simulink model "test_newfft_fun2"  (Simulink 6.2)
settings: Solver=ode45  StartTime=0.0  StopTime=3200.0  RelTol=1e-3
libraries: xbsIndex_r3 x643, simulink x1
(part 4 of 10)

== system test_newfft_fun2/r2_dit_fft/r2_dit_stage_5 ==
  a_in : Inport  Port=1  LatchInput=off
  b_in : Inport  Port=2  LatchInput=off
  sync_in : Inport  Port=3  LatchInput=off
  biplex_commutator : Subsystem  mask(Biplex Commutator){log2_size=6, n_bits=12, use_bram=off}
      mask prompts: log2_size "Log2 Block Size"; n_bits "Bit Width"; use_bram "Use BRAM"
      mask help: The biplex commutator commutes the first half of the BloBhi input "block" with the last half of the AloAhi input "block". A "block" is 2^log2_size consecutive samples (i.e. always a power of 2). sync_in precedes the first data input sample by one clock cycle. Overall latency from sync_in to sync_out is 2^(log2_size-1)+1.
      settings: AttributesFormatString=|
      | size = 64
      | delay slr
      mask Help:
      | <pre>
      | Description::
      | 
      | The biplex commutator commutes the first half of the BloBhi input "block"  with the last half
      | of the AloAhi input "block".  A "block" is 2^log2_size consecutive samples (i.e. always a
      | power of 2).
      | 
      | sync_in precedes the first data input sample by one clock cycle.
      | sync_out precedes the corresponding output sample by one clock cycle.
      | Overall latency from sync_in to sync_out is 2^(N-1)+1.
      | 
      | Mask Parameters::
      | 
      | Log 2 Block Size (log2_size): The base-2 logarithm of the length of one complete input block.
      | This MUST be an integer because the current implementation requires that
      | the input block size MUST be a power of 2.  (aka "N")
      | 
      | Bit Width (n_bits): Specifies the width of the real/imaginary components.
      | Width of each component is assumed equal.
      | 
      | Use BRAM (use_bram): Check this checkbox to implement the internal delays using BRAM.
      | If unchecked, the internal delays will be implemented using SLR16 elements.
      | </pre>
  r2_butterfly : Subsystem  mask(Radix-2 Butterfly){n_bits=12, shift=0, quantization=Truncate, add_latency=1}
      mask prompts: n_bits "Bit Width In"; shift "Shift Bits"; add_latency "Adder Latency"
      mask help: The radix-2 butterfly produces a+b and a-b outputs for a and b inputs.
      settings: AttributesFormatString=shift 0
      mask Help:
      | <pre>
      | Description::
      | 
      | The radix-2 butterfly produces a+b and a-b outputs for a and b inputs.
      | The outputs are one bit wider than the inputs.
      | The output precision (i.e. the number of fractional bits) stays the same.
      | 
      | Mask Parameters::
      | 
      | Bit Width In (n_bits): Specifies the width of the real/imaginary components.
      | Width of each component is assumed equal.
      | 
      | Shift Bits (shift): Specifies how many bits to shift (down) by.  A positive value causes
      | the specified number of least significant bits to be dropped.  Usually zero or positive values
      | are used to permit or limit bit growth, but negative values can be used to induce bit growth.
      | 
      | Quantization (quantization): Specifies quantization handling (when shift bits > 0).
      | 
      | Adder Latency (add_latency): Latency to use for the underlying real adders.
      | </pre>
      mask StyleString: edit,edit,popup(Truncate|Round  (unbiased: +/- Inf)|Round  (unbiased: Even Values)),edit
  r2_twiddle : Subsystem  mask(Radix-2 General Twiddle Stage){n_stages=10, cur_stage=5, decimation=Time, n_bits=12, bin_pt=7, n_bits_w=8, use_bram=off, mult_latency=3, add_latency=1}
      mask prompts: n_stages "Total Stages"; cur_stage "Current Stage"; decimation "Decimation Mode"; n_bits "Number of Bits In/Out"; bin_pt "Binary Point In/Out"; n_bits_w "Twiddle Coefficient Bitwidth"; use_bram "Use BRAM For Twiddle Coefficients"; mult_latency "Multiplier Latency"; add_latency "Adder Latency"
      mask help: A general twiddle stage for radix-2 Fast Fourier Transforms. Can be used in Decimation in Time (i.e. twiddles before butterflies) or Decimation in Frequency (i.e. twiddles after butterflies) FFTs. Regardless of the decimation mode, the FFT is assumed to have inputs in normal order and outputs in bit-reversed order.
      settings: AttributesFormatString=16 twiddles in dist
      mask Help:
      | <pre>
      | Description::
      | 
      | A general twiddle stage for radix-2 Fast Fourier Transforms.
      | 
      | Can be used in  Decimation in Time (i.e. twiddles before butterflies) or Decimation in Frequency
      | (i.e. twiddles after butterflies) FFTs.  Regardless of the decimation mode, the FFT is assumed
      | to have inputs in normal order and outputs in bit-reversed order.
      | 
      | Input a_in is passed through unchanged to a_out, while input b is passed through to bw after
      | being "twiddled".  Since twiddling is effectively multiplication by a complex number with unity
      | magnitude, the bit respresentation of bw is the same as b (i.e. twiddling does not cause bit
      | growth).  Input a_in is assumed to have the same bit width as b.  Thus, a_in, a_out, b, and
      | bw all have the same bit representation.
      | 
      | Mask Parameters::
      | 
      | Total Stages (n_stages):  The number of total stages in the FFT.
      | The FFT will have 2^n_stages points.
      | 
      | Current Stage (cur_stage):  The number of the current stage for which this block should
      | generate twiddle coefficients.  Valid values are 3 through n_stages, inclusive.  Note that
      | stages are counted from 1 to n_stages for DIT (i.e. cur_stage==1 for the first stage) and
      | n_stages to 1 for DIF (i.e. cur_stage==1 for the last stage).
      | 
      | Decimation Mode (decimation): The decimation mode of the FFT.
      | 
      | Number of Bits In/Out (n_bits): Specifies the width of the real/imaginary
      | components of ports a_in, b, a_out, bw.  Assumed equal for both components.
      | 
      | Binary Point In/Out (bin_pt): Specifies the binary point position of the real/imaginary
      | components of ports a_in, b, a_out, bw.  Assumed equal for both components.
      | 
      | Twiddle Coefficient Bitwidth (n_bits_w): Specifies the width of the real/imaginary
      | components of the twiddle coefficients.  Assumed equal for both components.
      | 
      | Use BRAM for Twiddle Coefficients (use_bram): Check this checkbox to store twiddle
      | coefficients in BRAM.  If unchecked, the twiddle coefficients will be sored in distributed
      | memory (i.e. slices).
      | 
      | Multiplier Latency (mult_latency): Latency to use for the underlying real multipliers.
      | 
      | Adder Latency (add_latency): Latency to use for the underlying real adders.
      mask StyleString: edit,edit,popup(Time|Frequency),edit,edit,edit,checkbox,edit,edit
  a_out : Outport
  b_out : Outport  Port=2
  sync_out : Outport  Port=3
  wires:
  r2_butterfly/3(sync_out) -> sync_out/1
  r2_butterfly/2(a-b) -> b_out/1
  r2_butterfly/1(a+b) -> a_out/1
  sync_in/1 -> biplex_commutator/3(sync_in)
  b_in/1 -> biplex_commutator/2(BloBhi)
  a_in/1 -> biplex_commutator/1(AloAhi)
  biplex_commutator/3(sync_out) -> r2_twiddle/3(sync_in)
  biplex_commutator/2(AhiBhi) -> r2_twiddle/2(b)
  biplex_commutator/1(AloBlo) -> r2_twiddle/1(a_in)
  r2_twiddle/1(a_out) -> r2_butterfly/1(a)
  r2_twiddle/2(bw) -> r2_butterfly/2(b)
  r2_twiddle/3(sync_out) -> r2_butterfly/3(sync_in)

== system test_newfft_fun2/r2_dit_fft/r2_dit_stage_6 ==
  a_in : Inport  Port=1  LatchInput=off
  b_in : Inport  Port=2  LatchInput=off
  sync_in : Inport  Port=3  LatchInput=off
  biplex_commutator : Subsystem  mask(Biplex Commutator){log2_size=5, n_bits=13, use_bram=off}
      mask prompts: log2_size "Log2 Block Size"; n_bits "Bit Width"; use_bram "Use BRAM"
      mask help: The biplex commutator commutes the first half of the BloBhi input "block" with the last half of the AloAhi input "block". A "block" is 2^log2_size consecutive samples (i.e. always a power of 2). sync_in precedes the first data input sample by one clock cycle. Overall latency from sync_in to sync_out is 2^(log2_size-1)+1.
      settings: AttributesFormatString=|
      | size = 32
      | delay slr
      mask Help:
      | <pre>
      | Description::
      | 
      | The biplex commutator commutes the first half of the BloBhi input "block"  with the last half
      | of the AloAhi input "block".  A "block" is 2^log2_size consecutive samples (i.e. always a
      | power of 2).
      | 
      | sync_in precedes the first data input sample by one clock cycle.
      | sync_out precedes the corresponding output sample by one clock cycle.
      | Overall latency from sync_in to sync_out is 2^(N-1)+1.
      | 
      | Mask Parameters::
      | 
      | Log 2 Block Size (log2_size): The base-2 logarithm of the length of one complete input block.
      | This MUST be an integer because the current implementation requires that
      | the input block size MUST be a power of 2.  (aka "N")
      | 
      | Bit Width (n_bits): Specifies the width of the real/imaginary components.
      | Width of each component is assumed equal.
      | 
      | Use BRAM (use_bram): Check this checkbox to implement the internal delays using BRAM.
      | If unchecked, the internal delays will be implemented using SLR16 elements.
      | </pre>
  r2_butterfly : Subsystem  mask(Radix-2 Butterfly){n_bits=13, shift=0, quantization=Truncate, add_latency=1}
      mask prompts: n_bits "Bit Width In"; shift "Shift Bits"; add_latency "Adder Latency"
      mask help: The radix-2 butterfly produces a+b and a-b outputs for a and b inputs.
      settings: AttributesFormatString=shift 0
      mask Help:
      | <pre>
      | Description::
      | 
      | The radix-2 butterfly produces a+b and a-b outputs for a and b inputs.
      | The outputs are one bit wider than the inputs.
      | The output precision (i.e. the number of fractional bits) stays the same.
      | 
      | Mask Parameters::
      | 
      | Bit Width In (n_bits): Specifies the width of the real/imaginary components.
      | Width of each component is assumed equal.
      | 
      | Shift Bits (shift): Specifies how many bits to shift (down) by.  A positive value causes
      | the specified number of least significant bits to be dropped.  Usually zero or positive values
      | are used to permit or limit bit growth, but negative values can be used to induce bit growth.
      | 
      | Quantization (quantization): Specifies quantization handling (when shift bits > 0).
      | 
      | Adder Latency (add_latency): Latency to use for the underlying real adders.
      | </pre>
      mask StyleString: edit,edit,popup(Truncate|Round  (unbiased: +/- Inf)|Round  (unbiased: Even Values)),edit
  r2_twiddle : Subsystem  mask(Radix-2 General Twiddle Stage){n_stages=10, cur_stage=6, decimation=Time, n_bits=13, bin_pt=7, n_bits_w=8, use_bram=off, mult_latency=3, add_latency=1}
      mask prompts: n_stages "Total Stages"; cur_stage "Current Stage"; decimation "Decimation Mode"; n_bits "Number of Bits In/Out"; bin_pt "Binary Point In/Out"; n_bits_w "Twiddle Coefficient Bitwidth"; use_bram "Use BRAM For Twiddle Coefficients"; mult_latency "Multiplier Latency"; add_latency "Adder Latency"
      mask help: A general twiddle stage for radix-2 Fast Fourier Transforms. Can be used in Decimation in Time (i.e. twiddles before butterflies) or Decimation in Frequency (i.e. twiddles after butterflies) FFTs. Regardless of the decimation mode, the FFT is assumed to have inputs in normal order and outputs in bit-reversed order.
      settings: AttributesFormatString=32 twiddles in dist
      mask Help:
      | <pre>
      | Description::
      | 
      | A general twiddle stage for radix-2 Fast Fourier Transforms.
      | 
      | Can be used in  Decimation in Time (i.e. twiddles before butterflies) or Decimation in Frequency
      | (i.e. twiddles after butterflies) FFTs.  Regardless of the decimation mode, the FFT is assumed
      | to have inputs in normal order and outputs in bit-reversed order.
      | 
      | Input a_in is passed through unchanged to a_out, while input b is passed through to bw after
      | being "twiddled".  Since twiddling is effectively multiplication by a complex number with unity
      | magnitude, the bit respresentation of bw is the same as b (i.e. twiddling does not cause bit
      | growth).  Input a_in is assumed to have the same bit width as b.  Thus, a_in, a_out, b, and
      | bw all have the same bit representation.
      | 
      | Mask Parameters::
      | 
      | Total Stages (n_stages):  The number of total stages in the FFT.
      | The FFT will have 2^n_stages points.
      | 
      | Current Stage (cur_stage):  The number of the current stage for which this block should
      | generate twiddle coefficients.  Valid values are 3 through n_stages, inclusive.  Note that
      | stages are counted from 1 to n_stages for DIT (i.e. cur_stage==1 for the first stage) and
      | n_stages to 1 for DIF (i.e. cur_stage==1 for the last stage).
      | 
      | Decimation Mode (decimation): The decimation mode of the FFT.
      | 
      | Number of Bits In/Out (n_bits): Specifies the width of the real/imaginary
      | components of ports a_in, b, a_out, bw.  Assumed equal for both components.
      | 
      | Binary Point In/Out (bin_pt): Specifies the binary point position of the real/imaginary
      | components of ports a_in, b, a_out, bw.  Assumed equal for both components.
      | 
      | Twiddle Coefficient Bitwidth (n_bits_w): Specifies the width of the real/imaginary
      | components of the twiddle coefficients.  Assumed equal for both components.
      | 
      | Use BRAM for Twiddle Coefficients (use_bram): Check this checkbox to store twiddle
      | coefficients in BRAM.  If unchecked, the twiddle coefficients will be sored in distributed
      | memory (i.e. slices).
      | 
      | Multiplier Latency (mult_latency): Latency to use for the underlying real multipliers.
      | 
      | Adder Latency (add_latency): Latency to use for the underlying real adders.
      mask StyleString: edit,edit,popup(Time|Frequency),edit,edit,edit,checkbox,edit,edit
  a_out : Outport
  b_out : Outport  Port=2
  sync_out : Outport  Port=3
  wires:
  r2_butterfly/3(sync_out) -> sync_out/1
  r2_butterfly/2(a-b) -> b_out/1
  r2_butterfly/1(a+b) -> a_out/1
  sync_in/1 -> biplex_commutator/3(sync_in)
  b_in/1 -> biplex_commutator/2(BloBhi)
  a_in/1 -> biplex_commutator/1(AloAhi)
  biplex_commutator/3(sync_out) -> r2_twiddle/3(sync_in)
  biplex_commutator/2(AhiBhi) -> r2_twiddle/2(b)
  biplex_commutator/1(AloBlo) -> r2_twiddle/1(a_in)
  r2_twiddle/1(a_out) -> r2_butterfly/1(a)
  r2_twiddle/2(bw) -> r2_butterfly/2(b)
  r2_twiddle/3(sync_out) -> r2_butterfly/3(sync_in)

== system test_newfft_fun2/r2_dit_fft/r2_dit_stage_7 ==
  a_in : Inport  Port=1  LatchInput=off
  b_in : Inport  Port=2  LatchInput=off
  sync_in : Inport  Port=3  LatchInput=off
  biplex_commutator : Subsystem  mask(Biplex Commutator){log2_size=4, n_bits=14, use_bram=off}
      mask prompts: log2_size "Log2 Block Size"; n_bits "Bit Width"; use_bram "Use BRAM"
      mask help: The biplex commutator commutes the first half of the BloBhi input "block" with the last half of the AloAhi input "block". A "block" is 2^log2_size consecutive samples (i.e. always a power of 2). sync_in precedes the first data input sample by one clock cycle. Overall latency from sync_in to sync_out is 2^(log2_size-1)+1.
      settings: AttributesFormatString=|
      | size = 16
      | delay slr
      mask Help:
      | <pre>
      | Description::
      | 
      | The biplex commutator commutes the first half of the BloBhi input "block"  with the last half
      | of the AloAhi input "block".  A "block" is 2^log2_size consecutive samples (i.e. always a
      | power of 2).
      | 
      | sync_in precedes the first data input sample by one clock cycle.
      | sync_out precedes the corresponding output sample by one clock cycle.
      | Overall latency from sync_in to sync_out is 2^(N-1)+1.
      | 
      | Mask Parameters::
      | 
      | Log 2 Block Size (log2_size): The base-2 logarithm of the length of one complete input block.
      | This MUST be an integer because the current implementation requires that
      | the input block size MUST be a power of 2.  (aka "N")
      | 
      | Bit Width (n_bits): Specifies the width of the real/imaginary components.
      | Width of each component is assumed equal.
      | 
      | Use BRAM (use_bram): Check this checkbox to implement the internal delays using BRAM.
      | If unchecked, the internal delays will be implemented using SLR16 elements.
      | </pre>
  r2_butterfly : Subsystem  mask(Radix-2 Butterfly){n_bits=14, shift=0, quantization=Truncate, add_latency=1}
      mask prompts: n_bits "Bit Width In"; shift "Shift Bits"; add_latency "Adder Latency"
      mask help: The radix-2 butterfly produces a+b and a-b outputs for a and b inputs.
      settings: AttributesFormatString=shift 0
      mask Help:
      | <pre>
      | Description::
      | 
      | The radix-2 butterfly produces a+b and a-b outputs for a and b inputs.
      | The outputs are one bit wider than the inputs.
      | The output precision (i.e. the number of fractional bits) stays the same.
      | 
      | Mask Parameters::
      | 
      | Bit Width In (n_bits): Specifies the width of the real/imaginary components.
      | Width of each component is assumed equal.
      | 
      | Shift Bits (shift): Specifies how many bits to shift (down) by.  A positive value causes
      | the specified number of least significant bits to be dropped.  Usually zero or positive values
      | are used to permit or limit bit growth, but negative values can be used to induce bit growth.
      | 
      | Quantization (quantization): Specifies quantization handling (when shift bits > 0).
      | 
      | Adder Latency (add_latency): Latency to use for the underlying real adders.
      | </pre>
      mask StyleString: edit,edit,popup(Truncate|Round  (unbiased: +/- Inf)|Round  (unbiased: Even Values)),edit
  r2_twiddle : Subsystem  mask(Radix-2 General Twiddle Stage){n_stages=10, cur_stage=7, decimation=Time, n_bits=14, bin_pt=7, n_bits_w=8, use_bram=off, mult_latency=3, add_latency=1}
      mask prompts: n_stages "Total Stages"; cur_stage "Current Stage"; decimation "Decimation Mode"; n_bits "Number of Bits In/Out"; bin_pt "Binary Point In/Out"; n_bits_w "Twiddle Coefficient Bitwidth"; use_bram "Use BRAM For Twiddle Coefficients"; mult_latency "Multiplier Latency"; add_latency "Adder Latency"
      mask help: A general twiddle stage for radix-2 Fast Fourier Transforms. Can be used in Decimation in Time (i.e. twiddles before butterflies) or Decimation in Frequency (i.e. twiddles after butterflies) FFTs. Regardless of the decimation mode, the FFT is assumed to have inputs in normal order and outputs in bit-reversed order.
      settings: AttributesFormatString=64 twiddles in dist
      mask Help:
      | <pre>
      | Description::
      | 
      | A general twiddle stage for radix-2 Fast Fourier Transforms.
      | 
      | Can be used in  Decimation in Time (i.e. twiddles before butterflies) or Decimation in Frequency
      | (i.e. twiddles after butterflies) FFTs.  Regardless of the decimation mode, the FFT is assumed
      | to have inputs in normal order and outputs in bit-reversed order.
      | 
      | Input a_in is passed through unchanged to a_out, while input b is passed through to bw after
      | being "twiddled".  Since twiddling is effectively multiplication by a complex number with unity
      | magnitude, the bit respresentation of bw is the same as b (i.e. twiddling does not cause bit
      | growth).  Input a_in is assumed to have the same bit width as b.  Thus, a_in, a_out, b, and
      | bw all have the same bit representation.
      | 
      | Mask Parameters::
      | 
      | Total Stages (n_stages):  The number of total stages in the FFT.
      | The FFT will have 2^n_stages points.
      | 
      | Current Stage (cur_stage):  The number of the current stage for which this block should
      | generate twiddle coefficients.  Valid values are 3 through n_stages, inclusive.  Note that
      | stages are counted from 1 to n_stages for DIT (i.e. cur_stage==1 for the first stage) and
      | n_stages to 1 for DIF (i.e. cur_stage==1 for the last stage).
      | 
      | Decimation Mode (decimation): The decimation mode of the FFT.
      | 
      | Number of Bits In/Out (n_bits): Specifies the width of the real/imaginary
      | components of ports a_in, b, a_out, bw.  Assumed equal for both components.
      | 
      | Binary Point In/Out (bin_pt): Specifies the binary point position of the real/imaginary
      | components of ports a_in, b, a_out, bw.  Assumed equal for both components.
      | 
      | Twiddle Coefficient Bitwidth (n_bits_w): Specifies the width of the real/imaginary
      | components of the twiddle coefficients.  Assumed equal for both components.
      | 
      | Use BRAM for Twiddle Coefficients (use_bram): Check this checkbox to store twiddle
      | coefficients in BRAM.  If unchecked, the twiddle coefficients will be sored in distributed
      | memory (i.e. slices).
      | 
      | Multiplier Latency (mult_latency): Latency to use for the underlying real multipliers.
      | 
      | Adder Latency (add_latency): Latency to use for the underlying real adders.
      mask StyleString: edit,edit,popup(Time|Frequency),edit,edit,edit,checkbox,edit,edit
  a_out : Outport
  b_out : Outport  Port=2
  sync_out : Outport  Port=3
  wires:
  r2_butterfly/3(sync_out) -> sync_out/1
  r2_butterfly/2(a-b) -> b_out/1
  r2_butterfly/1(a+b) -> a_out/1
  sync_in/1 -> biplex_commutator/3(sync_in)
  b_in/1 -> biplex_commutator/2(BloBhi)
  a_in/1 -> biplex_commutator/1(AloAhi)
  biplex_commutator/3(sync_out) -> r2_twiddle/3(sync_in)
  biplex_commutator/2(AhiBhi) -> r2_twiddle/2(b)
  biplex_commutator/1(AloBlo) -> r2_twiddle/1(a_in)
  r2_twiddle/1(a_out) -> r2_butterfly/1(a)
  r2_twiddle/2(bw) -> r2_butterfly/2(b)
  r2_twiddle/3(sync_out) -> r2_butterfly/3(sync_in)

== system test_newfft_fun2/r2_dit_fft/r2_dit_stage_8 ==
  a_in : Inport  Port=1  LatchInput=off
  b_in : Inport  Port=2  LatchInput=off
  sync_in : Inport  Port=3  LatchInput=off
  biplex_commutator : Subsystem  mask(Biplex Commutator){log2_size=3, n_bits=15, use_bram=off}
      mask prompts: log2_size "Log2 Block Size"; n_bits "Bit Width"; use_bram "Use BRAM"
      mask help: The biplex commutator commutes the first half of the BloBhi input "block" with the last half of the AloAhi input "block". A "block" is 2^log2_size consecutive samples (i.e. always a power of 2). sync_in precedes the first data input sample by one clock cycle. Overall latency from sync_in to sync_out is 2^(log2_size-1)+1.
      settings: AttributesFormatString=|
      | size = 8
      | delay slr
      mask Help:
      | <pre>
      | Description::
      | 
      | The biplex commutator commutes the first half of the BloBhi input "block"  with the last half
      | of the AloAhi input "block".  A "block" is 2^log2_size consecutive samples (i.e. always a
      | power of 2).
      | 
      | sync_in precedes the first data input sample by one clock cycle.
      | sync_out precedes the corresponding output sample by one clock cycle.
      | Overall latency from sync_in to sync_out is 2^(N-1)+1.
      | 
      | Mask Parameters::
      | 
      | Log 2 Block Size (log2_size): The base-2 logarithm of the length of one complete input block.
      | This MUST be an integer because the current implementation requires that
      | the input block size MUST be a power of 2.  (aka "N")
      | 
      | Bit Width (n_bits): Specifies the width of the real/imaginary components.
      | Width of each component is assumed equal.
      | 
      | Use BRAM (use_bram): Check this checkbox to implement the internal delays using BRAM.
      | If unchecked, the internal delays will be implemented using SLR16 elements.
      | </pre>
  r2_butterfly : Subsystem  mask(Radix-2 Butterfly){n_bits=15, shift=0, quantization=Truncate, add_latency=1}
      mask prompts: n_bits "Bit Width In"; shift "Shift Bits"; add_latency "Adder Latency"
      mask help: The radix-2 butterfly produces a+b and a-b outputs for a and b inputs.
      settings: AttributesFormatString=shift 0
      mask Help:
      | <pre>
      | Description::
      | 
      | The radix-2 butterfly produces a+b and a-b outputs for a and b inputs.
      | The outputs are one bit wider than the inputs.
      | The output precision (i.e. the number of fractional bits) stays the same.
      | 
      | Mask Parameters::
      | 
      | Bit Width In (n_bits): Specifies the width of the real/imaginary components.
      | Width of each component is assumed equal.
      | 
      | Shift Bits (shift): Specifies how many bits to shift (down) by.  A positive value causes
      | the specified number of least significant bits to be dropped.  Usually zero or positive values
      | are used to permit or limit bit growth, but negative values can be used to induce bit growth.
      | 
      | Quantization (quantization): Specifies quantization handling (when shift bits > 0).
      | 
      | Adder Latency (add_latency): Latency to use for the underlying real adders.
      | </pre>
      mask StyleString: edit,edit,popup(Truncate|Round  (unbiased: +/- Inf)|Round  (unbiased: Even Values)),edit
  r2_twiddle : Subsystem  mask(Radix-2 General Twiddle Stage){n_stages=10, cur_stage=8, decimation=Time, n_bits=15, bin_pt=7, n_bits_w=8, use_bram=off, mult_latency=3, add_latency=1}
      mask prompts: n_stages "Total Stages"; cur_stage "Current Stage"; decimation "Decimation Mode"; n_bits "Number of Bits In/Out"; bin_pt "Binary Point In/Out"; n_bits_w "Twiddle Coefficient Bitwidth"; use_bram "Use BRAM For Twiddle Coefficients"; mult_latency "Multiplier Latency"; add_latency "Adder Latency"
      mask help: A general twiddle stage for radix-2 Fast Fourier Transforms. Can be used in Decimation in Time (i.e. twiddles before butterflies) or Decimation in Frequency (i.e. twiddles after butterflies) FFTs. Regardless of the decimation mode, the FFT is assumed to have inputs in normal order and outputs in bit-reversed order.
      settings: AttributesFormatString=128 twiddles in dist
      mask Help:
      | <pre>
      | Description::
      | 
      | A general twiddle stage for radix-2 Fast Fourier Transforms.
      | 
      | Can be used in  Decimation in Time (i.e. twiddles before butterflies) or Decimation in Frequency
      | (i.e. twiddles after butterflies) FFTs.  Regardless of the decimation mode, the FFT is assumed
      | to have inputs in normal order and outputs in bit-reversed order.
      | 
      | Input a_in is passed through unchanged to a_out, while input b is passed through to bw after
      | being "twiddled".  Since twiddling is effectively multiplication by a complex number with unity
      | magnitude, the bit respresentation of bw is the same as b (i.e. twiddling does not cause bit
      | growth).  Input a_in is assumed to have the same bit width as b.  Thus, a_in, a_out, b, and
      | bw all have the same bit representation.
      | 
      | Mask Parameters::
      | 
      | Total Stages (n_stages):  The number of total stages in the FFT.
      | The FFT will have 2^n_stages points.
      | 
      | Current Stage (cur_stage):  The number of the current stage for which this block should
      | generate twiddle coefficients.  Valid values are 3 through n_stages, inclusive.  Note that
      | stages are counted from 1 to n_stages for DIT (i.e. cur_stage==1 for the first stage) and
      | n_stages to 1 for DIF (i.e. cur_stage==1 for the last stage).
      | 
      | Decimation Mode (decimation): The decimation mode of the FFT.
      | 
      | Number of Bits In/Out (n_bits): Specifies the width of the real/imaginary
      | components of ports a_in, b, a_out, bw.  Assumed equal for both components.
      | 
      | Binary Point In/Out (bin_pt): Specifies the binary point position of the real/imaginary
      | components of ports a_in, b, a_out, bw.  Assumed equal for both components.
      | 
      | Twiddle Coefficient Bitwidth (n_bits_w): Specifies the width of the real/imaginary
      | components of the twiddle coefficients.  Assumed equal for both components.
      | 
      | Use BRAM for Twiddle Coefficients (use_bram): Check this checkbox to store twiddle
      | coefficients in BRAM.  If unchecked, the twiddle coefficients will be sored in distributed
      | memory (i.e. slices).
      | 
      | Multiplier Latency (mult_latency): Latency to use for the underlying real multipliers.
      | 
      | Adder Latency (add_latency): Latency to use for the underlying real adders.
      mask StyleString: edit,edit,popup(Time|Frequency),edit,edit,edit,checkbox,edit,edit
  a_out : Outport
  b_out : Outport  Port=2
  sync_out : Outport  Port=3
  wires:
  r2_butterfly/3(sync_out) -> sync_out/1
  r2_butterfly/2(a-b) -> b_out/1
  r2_butterfly/1(a+b) -> a_out/1
  sync_in/1 -> biplex_commutator/3(sync_in)
  b_in/1 -> biplex_commutator/2(BloBhi)
  a_in/1 -> biplex_commutator/1(AloAhi)
  biplex_commutator/3(sync_out) -> r2_twiddle/3(sync_in)
  biplex_commutator/2(AhiBhi) -> r2_twiddle/2(b)
  biplex_commutator/1(AloBlo) -> r2_twiddle/1(a_in)
  r2_twiddle/1(a_out) -> r2_butterfly/1(a)
  r2_twiddle/2(bw) -> r2_butterfly/2(b)
  r2_twiddle/3(sync_out) -> r2_butterfly/3(sync_in)

== system test_newfft_fun2/r2_dit_fft/r2_dit_stage_9 ==
  a_in : Inport  Port=1  LatchInput=off
  b_in : Inport  Port=2  LatchInput=off
  sync_in : Inport  Port=3  LatchInput=off
  biplex_commutator : Subsystem  mask(Biplex Commutator){log2_size=2, n_bits=16, use_bram=off}
      mask prompts: log2_size "Log2 Block Size"; n_bits "Bit Width"; use_bram "Use BRAM"
      mask help: The biplex commutator commutes the first half of the BloBhi input "block" with the last half of the AloAhi input "block". A "block" is 2^log2_size consecutive samples (i.e. always a power of 2). sync_in precedes the first data input sample by one clock cycle. Overall latency from sync_in to sync_out is 2^(log2_size-1)+1.
      settings: AttributesFormatString=|
      | size = 4
      | delay slr
      mask Help:
      | <pre>
      | Description::
      | 
      | The biplex commutator commutes the first half of the BloBhi input "block"  with the last half
      | of the AloAhi input "block".  A "block" is 2^log2_size consecutive samples (i.e. always a
      | power of 2).
      | 
      | sync_in precedes the first data input sample by one clock cycle.
      | sync_out precedes the corresponding output sample by one clock cycle.
      | Overall latency from sync_in to sync_out is 2^(N-1)+1.
      | 
      | Mask Parameters::
      | 
      | Log 2 Block Size (log2_size): The base-2 logarithm of the length of one complete input block.
      | This MUST be an integer because the current implementation requires that
      | the input block size MUST be a power of 2.  (aka "N")
      | 
      | Bit Width (n_bits): Specifies the width of the real/imaginary components.
      | Width of each component is assumed equal.
      | 
      | Use BRAM (use_bram): Check this checkbox to implement the internal delays using BRAM.
      | If unchecked, the internal delays will be implemented using SLR16 elements.
      | </pre>
  r2_butterfly : Subsystem  mask(Radix-2 Butterfly){n_bits=16, shift=0, quantization=Truncate, add_latency=1}
      mask prompts: n_bits "Bit Width In"; shift "Shift Bits"; add_latency "Adder Latency"
      mask help: The radix-2 butterfly produces a+b and a-b outputs for a and b inputs.
      settings: AttributesFormatString=shift 0
      mask Help:
      | <pre>
      | Description::
      | 
      | The radix-2 butterfly produces a+b and a-b outputs for a and b inputs.
      | The outputs are one bit wider than the inputs.
      | The output precision (i.e. the number of fractional bits) stays the same.
      | 
      | Mask Parameters::
      | 
      | Bit Width In (n_bits): Specifies the width of the real/imaginary components.
      | Width of each component is assumed equal.
      | 
      | Shift Bits (shift): Specifies how many bits to shift (down) by.  A positive value causes
      | the specified number of least significant bits to be dropped.  Usually zero or positive values
      | are used to permit or limit bit growth, but negative values can be used to induce bit growth.
      | 
      | Quantization (quantization): Specifies quantization handling (when shift bits > 0).
      | 
      | Adder Latency (add_latency): Latency to use for the underlying real adders.
      | </pre>
      mask StyleString: edit,edit,popup(Truncate|Round  (unbiased: +/- Inf)|Round  (unbiased: Even Values)),edit
  r2_twiddle : Subsystem  mask(Radix-2 General Twiddle Stage){n_stages=10, cur_stage=9, decimation=Time, n_bits=16, bin_pt=7, n_bits_w=8, use_bram=off, mult_latency=3, add_latency=1}
      mask prompts: n_stages "Total Stages"; cur_stage "Current Stage"; decimation "Decimation Mode"; n_bits "Number of Bits In/Out"; bin_pt "Binary Point In/Out"; n_bits_w "Twiddle Coefficient Bitwidth"; use_bram "Use BRAM For Twiddle Coefficients"; mult_latency "Multiplier Latency"; add_latency "Adder Latency"
      mask help: A general twiddle stage for radix-2 Fast Fourier Transforms. Can be used in Decimation in Time (i.e. twiddles before butterflies) or Decimation in Frequency (i.e. twiddles after butterflies) FFTs. Regardless of the decimation mode, the FFT is assumed to have inputs in normal order and outputs in bit-reversed order.
      settings: AttributesFormatString=256 twiddles in dist
      mask Help:
      | <pre>
      | Description::
      | 
      | A general twiddle stage for radix-2 Fast Fourier Transforms.
      | 
      | Can be used in  Decimation in Time (i.e. twiddles before butterflies) or Decimation in Frequency
      | (i.e. twiddles after butterflies) FFTs.  Regardless of the decimation mode, the FFT is assumed
      | to have inputs in normal order and outputs in bit-reversed order.
      | 
      | Input a_in is passed through unchanged to a_out, while input b is passed through to bw after
      | being "twiddled".  Since twiddling is effectively multiplication by a complex number with unity
      | magnitude, the bit respresentation of bw is the same as b (i.e. twiddling does not cause bit
      | growth).  Input a_in is assumed to have the same bit width as b.  Thus, a_in, a_out, b, and
      | bw all have the same bit representation.
      | 
      | Mask Parameters::
      | 
      | Total Stages (n_stages):  The number of total stages in the FFT.
      | The FFT will have 2^n_stages points.
      | 
      | Current Stage (cur_stage):  The number of the current stage for which this block should
      | generate twiddle coefficients.  Valid values are 3 through n_stages, inclusive.  Note that
      | stages are counted from 1 to n_stages for DIT (i.e. cur_stage==1 for the first stage) and
      | n_stages to 1 for DIF (i.e. cur_stage==1 for the last stage).
      | 
      | Decimation Mode (decimation): The decimation mode of the FFT.
      | 
      | Number of Bits In/Out (n_bits): Specifies the width of the real/imaginary
      | components of ports a_in, b, a_out, bw.  Assumed equal for both components.
      | 
      | Binary Point In/Out (bin_pt): Specifies the binary point position of the real/imaginary
      | components of ports a_in, b, a_out, bw.  Assumed equal for both components.
      | 
      | Twiddle Coefficient Bitwidth (n_bits_w): Specifies the width of the real/imaginary
      | components of the twiddle coefficients.  Assumed equal for both components.
      | 
      | Use BRAM for Twiddle Coefficients (use_bram): Check this checkbox to store twiddle
      | coefficients in BRAM.  If unchecked, the twiddle coefficients will be sored in distributed
      | memory (i.e. slices).
      | 
      | Multiplier Latency (mult_latency): Latency to use for the underlying real multipliers.
      | 
      | Adder Latency (add_latency): Latency to use for the underlying real adders.
      mask StyleString: edit,edit,popup(Time|Frequency),edit,edit,edit,checkbox,edit,edit
  a_out : Outport
  b_out : Outport  Port=2
  sync_out : Outport  Port=3
  wires:
  r2_butterfly/3(sync_out) -> sync_out/1
  r2_butterfly/2(a-b) -> b_out/1
  r2_butterfly/1(a+b) -> a_out/1
  sync_in/1 -> biplex_commutator/3(sync_in)
  b_in/1 -> biplex_commutator/2(BloBhi)
  a_in/1 -> biplex_commutator/1(AloAhi)
  biplex_commutator/3(sync_out) -> r2_twiddle/3(sync_in)
  biplex_commutator/2(AhiBhi) -> r2_twiddle/2(b)
  biplex_commutator/1(AloBlo) -> r2_twiddle/1(a_in)
  r2_twiddle/1(a_out) -> r2_butterfly/1(a)
  r2_twiddle/2(bw) -> r2_butterfly/2(b)
  r2_twiddle/3(sync_out) -> r2_butterfly/3(sync_in)

== system test_newfft_fun2/r2_dit_fft/biplex_bitrev/bit_reverse ==
  in : Inport  Port=1  LatchInput=off
  bit0 : xbsIndex_r3/Slice  mode=Lower Bit Location + Width  nbits=1  bit1=0  base1=MSB of Input  bit0=0  base0=LSB of Input  boolean_output=off  explicit_period=off  period=1  dbl_ovrd=off
  bit1 : xbsIndex_r3/Slice  mode=Lower Bit Location + Width  nbits=1  bit1=0  base1=MSB of Input  bit0=1  base0=LSB of Input  boolean_output=off  explicit_period=off  period=1  dbl_ovrd=off
  bit2 : xbsIndex_r3/Slice  mode=Lower Bit Location + Width  nbits=1  bit1=0  base1=MSB of Input  bit0=2  base0=LSB of Input  boolean_output=off  explicit_period=off  period=1  dbl_ovrd=off
  bit3 : xbsIndex_r3/Slice  mode=Lower Bit Location + Width  nbits=1  bit1=0  base1=MSB of Input  bit0=3  base0=LSB of Input  boolean_output=off  explicit_period=off  period=1  dbl_ovrd=off
  bit4 : xbsIndex_r3/Slice  mode=Lower Bit Location + Width  nbits=1  bit1=0  base1=MSB of Input  bit0=4  base0=LSB of Input  boolean_output=off  explicit_period=off  period=1  dbl_ovrd=off
  bit5 : xbsIndex_r3/Slice  mode=Lower Bit Location + Width  nbits=1  bit1=0  base1=MSB of Input  bit0=5  base0=LSB of Input  boolean_output=off  explicit_period=off  period=1  dbl_ovrd=off
  bit6 : xbsIndex_r3/Slice  mode=Lower Bit Location + Width  nbits=1  bit1=0  base1=MSB of Input  bit0=6  base0=LSB of Input  boolean_output=off  explicit_period=off  period=1  dbl_ovrd=off
  bit7 : xbsIndex_r3/Slice  mode=Lower Bit Location + Width  nbits=1  bit1=0  base1=MSB of Input  bit0=7  base0=LSB of Input  boolean_output=off  explicit_period=off  period=1  dbl_ovrd=off
  bit8 : xbsIndex_r3/Slice  mode=Lower Bit Location + Width  nbits=1  bit1=0  base1=MSB of Input  bit0=8  base0=LSB of Input  boolean_output=off  explicit_period=off  period=1  dbl_ovrd=off
  concat : xbsIndex_r3/Concat  num_inputs=9  explicit_period=off  period=1  dbl_ovrd=off
  out : Outport
  wires:
  in/1 -> bit8/1, bit7/1, bit6/1, bit5/1, bit4/1, bit3/1, bit2/1, bit1/1, bit0/1
  bit8/1 -> concat/9
  bit7/1 -> concat/8
  bit6/1 -> concat/7
  bit5/1 -> concat/6
  bit4/1 -> concat/5
  bit3/1 -> concat/4
  bit2/1 -> concat/3
  bit1/1 -> concat/2
  bit0/1 -> concat/1
  concat/1 -> out/1

== system test_newfft_fun2/r2_dit_fft/biplex_bitrev/c_to_ri ==
  c : Inport  Port=1  LatchInput=off
  force_im : xbsIndex_r3/Reinterpret  force_arith_type=on  arith_type="Signed  (2's comp)"  force_bin_pt=on  bin_pt=0  force_valid=on
  force_re : xbsIndex_r3/Reinterpret  force_arith_type=on  arith_type="Signed  (2's comp)"  force_bin_pt=on  bin_pt=0  force_valid=on
  slice_im : xbsIndex_r3/Slice  mode=Lower Bit Location + Width  nbits=18  bit1=0  base1=MSB of Input  bit0=0  base0=LSB of Input  boolean_output=off  explicit_period=off  period=1  dbl_ovrd=off
  slice_re : xbsIndex_r3/Slice  mode=Upper Bit Location + Width  nbits=18  bit1=0  base1=MSB of Input  bit0=0  base0=LSB of Input  boolean_output=off  explicit_period=off  period=1  dbl_ovrd=off
  re : Outport
  im : Outport  Port=2
  wires:
  slice_re/1 -> force_re/1
  slice_im/1 -> force_im/1
  force_re/1 -> re/1
  force_im/1 -> im/1
  c/1 -> slice_re/1, slice_im/1

== system test_newfft_fun2/r2_dit_fft/biplex_bitrev/c_to_ri1 ==
  c : Inport  Port=1  LatchInput=off
  force_im : xbsIndex_r3/Reinterpret  force_arith_type=on  arith_type="Signed  (2's comp)"  force_bin_pt=on  bin_pt=0  force_valid=on
  force_re : xbsIndex_r3/Reinterpret  force_arith_type=on  arith_type="Signed  (2's comp)"  force_bin_pt=on  bin_pt=0  force_valid=on
  slice_im : xbsIndex_r3/Slice  mode=Lower Bit Location + Width  nbits=18  bit1=0  base1=MSB of Input  bit0=0  base0=LSB of Input  boolean_output=off  explicit_period=off  period=1  dbl_ovrd=off
  slice_re : xbsIndex_r3/Slice  mode=Upper Bit Location + Width  nbits=18  bit1=0  base1=MSB of Input  bit0=0  base0=LSB of Input  boolean_output=off  explicit_period=off  period=1  dbl_ovrd=off
  re : Outport
  im : Outport  Port=2
  wires:
  slice_re/1 -> force_re/1
  slice_im/1 -> force_im/1
  force_re/1 -> re/1
  force_im/1 -> im/1
  c/1 -> slice_re/1, slice_im/1

== system test_newfft_fun2/r2_dit_fft/biplex_bitrev/ri_to_c ==
  re : Inport  Port=1  LatchInput=off
  im : Inport  Port=2  LatchInput=off
  concat : xbsIndex_r3/Concat  num_inputs=2  explicit_period=off  period=1  dbl_ovrd=off
  force_im : xbsIndex_r3/Reinterpret  force_arith_type=on  arith_type=Unsigned  force_bin_pt=on  bin_pt=0  force_valid=on
  force_re : xbsIndex_r3/Reinterpret  force_arith_type=on  arith_type=Unsigned  force_bin_pt=on  bin_pt=0  force_valid=on
  c : Outport
  wires:
  force_re/1 -> concat/1
  force_im/1 -> concat/2
  re/1 -> force_re/1
  concat/1 -> c/1
  im/1 -> force_im/1

== system test_newfft_fun2/r2_dit_fft/biplex_bitrev/ri_to_c1 ==
  re : Inport  Port=1  LatchInput=off
  im : Inport  Port=2  LatchInput=off
  concat : xbsIndex_r3/Concat  num_inputs=2  explicit_period=off  period=1  dbl_ovrd=off
  force_im : xbsIndex_r3/Reinterpret  force_arith_type=on  arith_type=Unsigned  force_bin_pt=on  bin_pt=0  force_valid=on
  force_re : xbsIndex_r3/Reinterpret  force_arith_type=on  arith_type=Unsigned  force_bin_pt=on  bin_pt=0  force_valid=on
  c : Outport
  wires:
  force_re/1 -> concat/1
  force_im/1 -> concat/2
  re/1 -> force_re/1
  concat/1 -> c/1
  im/1 -> force_im/1

== system test_newfft_fun2/r2_dit_fft/biplex_commutator/delay_b ==
  in : Inport  Port=1  LatchInput=off
  slr : xbsIndex_r3/Delay  latency=512  reg_retiming=off  explicit_period=off  period=1  en=off  accept_only_valid=off  init_zero=on  dbl_ovrd=off  show_param=off
      settings: xl_area=[0, 0, 0, 0, 0, 0, 0]
  out : Outport
  wires:
  slr/1 -> out/1
  in/1 -> slr/1

== system test_newfft_fun2/r2_dit_fft/biplex_commutator/delay_lo ==
  in : Inport  Port=1  LatchInput=off
  slr : xbsIndex_r3/Delay  latency=512  reg_retiming=off  explicit_period=off  period=1  en=off  accept_only_valid=off  init_zero=on  dbl_ovrd=off  show_param=off
      settings: xl_area=[0, 0, 0, 0, 0, 0, 0]
  out : Outport
  wires:
  slr/1 -> out/1
  in/1 -> slr/1

== system test_newfft_fun2/r2_dit_fft/r2_dit_stage_1/biplex_commutator ==
  AloAhi : Inport  Port=1  LatchInput=off
  BloBhi : Inport  Port=2  LatchInput=off
  sync_in : Inport  Port=3  LatchInput=off
  Counter : xbsIndex_r3/Counter  cnt_type=Free Running  n_bits=10  bin_pt=0  arith_type=Unsigned  start_count=0  cnt_to=Inf  cnt_by_val=1  operation=Up  explicit_period=off  period=1  load_pin=off  rst=on  en=off  dbl_ovrd=off  show_param=off  use_rpm=on  gen_core=off
      settings: xl_area=[0, 0, 0, 0, 0, 0, 0]
  Delay : xbsIndex_r3/Delay  latency=513  reg_retiming=off  explicit_period=off  period=1  en=off  accept_only_valid=off  init_zero=on  dbl_ovrd=off  show_param=off
      settings: xl_area=[0, 0, 0, 0, 0, 0, 0]
  Mux : xbsIndex_r3/Mux  inputs=2  precision=Full  arith_type="Signed  (2's comp)"  n_bits=8  bin_pt=2  quantization=Truncate  overflow=Wrap  latency=1  explicit_period=off  period=1  en=off  dbl_ovrd=off  show_param=off  mux_type=off  use_rpm=off  gen_core=off
      settings: xl_area=[0, 0, 0, 0, 0, 0, 0]
  Mux1 : xbsIndex_r3/Mux  inputs=2  precision=Full  arith_type="Signed  (2's comp)"  n_bits=8  bin_pt=2  quantization=Truncate  overflow=Wrap  latency=1  explicit_period=off  period=1  en=off  dbl_ovrd=off  show_param=on  mux_type=off  use_rpm=off  gen_core=off
      settings: xl_area=[0, 0, 0, 0, 0, 0, 0]
  delay_b : Subsystem  mask(SLR16 Delay){delay_depth=512}
      mask prompts: delay_depth "Delay Depth"
      mask help: A delay block that uses SLR16 elements for its storage.
      settings: AttributesFormatString=slr depth = 512
      mask Help:
      | <pre>
      | Description::
      | 
      | A delay block that uses SLR16 elements for its storage.
      | 
      | Mask Parameters::
      | 
      | Delay Depth (delay_depth): The length of the delay.
      | </pre>
  delay_lo : Subsystem  mask(SLR16 Delay){delay_depth=512}
      mask prompts: delay_depth "Delay Depth"
      mask help: A delay block that uses SLR16 elements for its storage.
      settings: AttributesFormatString=slr depth = 512
      mask Help:
      | <pre>
      | Description::
      | 
      | A delay block that uses SLR16 elements for its storage.
      | 
      | Mask Parameters::
      | 
      | Delay Depth (delay_depth): The length of the delay.
      | </pre>
  top_bit : xbsIndex_r3/Slice  mode=Upper Bit Location + Width  nbits=1  bit1=0  base1=MSB of Input  bit0=0  base0=LSB of Input  boolean_output=off  explicit_period=off  period=1  dbl_ovrd=off
  AloBlo : Outport
  AhiBhi : Outport  Port=2
  sync_out : Outport  Port=3
  wires:
  Delay/1 -> sync_out/1
  delay_lo/1(out) -> AloBlo/1
  Mux/1 -> delay_lo/1(in)
  delay_b/1(out) -> Mux/3, Mux1/2
  BloBhi/1 -> delay_b/1(in)
  Mux1/1 -> AhiBhi/1
  AloAhi/1 -> Mux1/3, Mux/2
  top_bit/1 -> Mux/1, Mux1/1
  Counter/1 -> top_bit/1
  sync_in/1 -> Delay/1, Counter/1
